simulink model "hw2_DCM_constant_flux"  (R2022a)
settings: Solver=ode45  StartTime=0.0  StopTime=10  MaxStep=0.0001  RelTol=1e-3  EnableMultiTasking=on
values from neighbouring files (symbols this model uses):
  Fv = 0.01 + N/3000    (= 0.0236666666667)    [hw2.m]    (also in hw3.m)
  J = 0.46    [hw2.m]    (also in hw3.m)
  kfi = M/In    (= 4.56074766355)    [hw2.m]    (also in hw3.m)
  La = 0.007    [hw2.m]    (also in hw3.m = 0.0007)
  Ra = 0.578    [hw2.m]    (also in hw3.m)
undefined symbols (not defined in the file or in its folder): sigbuilder_block
libraries: simulink x2
settings Model: Creator=user  LastModifiedBy=geote
settings SolverCC: AlgebraicLoopSolver=TrustRegion
settings DataIOCC: LimitDataPoints=on  SaveFormat=Array  SignalLoggingSaveFormat=ModelDataLogs  ReturnWorkspaceOutputs=off  SignalLoggingName=sigsOut
settings OptimizationCC: ExpressionDepthLimit=2147483647  InitFltsAndDblsToZero=on  LifeSpan=inf
settings DebuggingCC: SaveWithParameterizedLinksMsg=none  UnderspecifiedInitializationDetection=Classic  MergeDetectMultiDrivingBlocksExec=none  SignalResolutionControl=TryResolveAllWithWarning  MultiTaskDSMMsg=warning  MultiTaskCondExecSysMsg=none  FcnCallInpInsideContextMsg=warning  UnconnectedInputMsg=warning  UnconnectedOutputMsg=warning  UnconnectedLineMsg=warning  StateNameClashWarn=warning  SFUnexpectedBacktrackingDiag=warning  SFNoUnconditionalDefaultTransitionDiag=warning  SFMachineParentedDataDiag=warning  ArithmeticOperatorsInVariantConditions=warning
settings HardwareCC: ProdBitPerPointer=32  ProdBitPerSizeT=32  ProdBitPerPtrDiffT=32  ProdLargestAtomicFloat=None  ProdIntDivRoundTo=Undefined  ProdEndianess=Unspecified  ProdWordSize=32  ProdHWDeviceType=32-bit Generic  TargetUnknown=on
settings ModelReferenceCC: PropagateSignalLabelsOutOfModel=off
settings SFSimCC: SimUseLocalCustomCode=off  CustomCodeUndefinedFunction=UseInterfaceOnly
settings RTWCC: RTWUseLocalCustomCode=off
settings CodeAppCC: StateflowObjectComments=on
settings GRTTargetCC: TargetFcnLib=ansi_tfl_tmw.mat  TargetLangStandard=C89/C90 (ANSI)  CombineOutputUpdateFcns=off  GRTInterface=on
settings ConfigComp: CovMetricSettings=dw  CovSaveCumulativeToWorkspaceVar=on  CovSaveSingleToWorkspaceVar=on  CovExternalEMLEnable=off

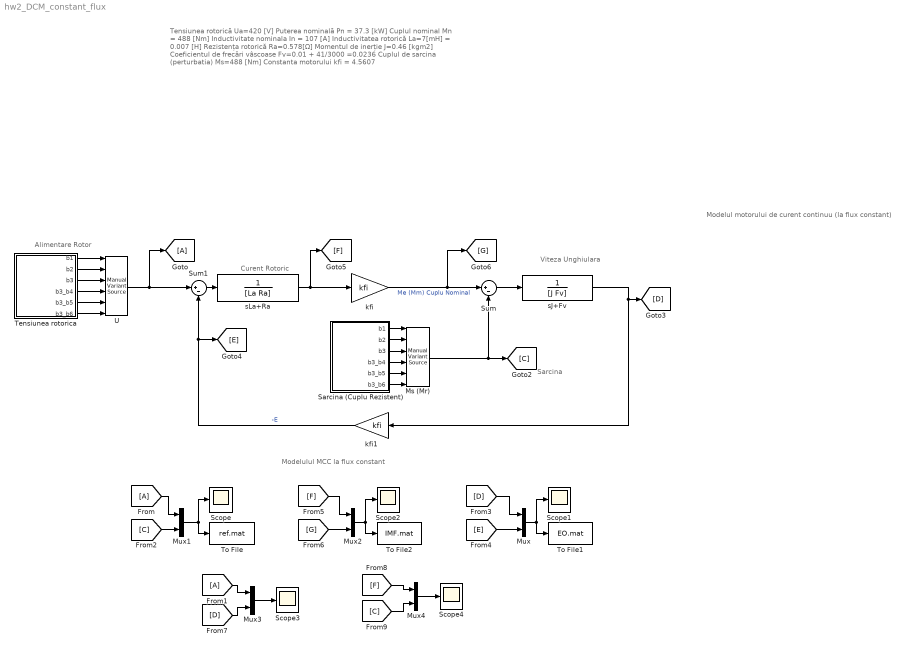
== system hw2_DCM_constant_flux ==
  note: Modelul motorului de curent continuu (la flux constant)
  note: Curent Rotoric
  note: Viteza
      | Unghiulara
  note: Modelulul MCC la flux constant
  note: Tensiunea rotorică Ua=420 [V]
      | Puterea nominală Pn = 37.3 [kW]
      |
      | Cuplul nominal Mn = 488 [Nm]
      | Inductivitate nominala In = 107 [A]
      |
      | Inductivitatea rotorică La=7[mH] = 0.007 [H]
      | Rezistența rotorică Ra=0.578[Ω]
      |
      | Momentul de inerție J=0.46 [kgm2]
      | Coeficientul de frecări vâscoase Fv=0.01 + 41/3000 =0.0236
      |
      | Cuplul de sarcina (perturbatia) Ms=488 [Nm]
      |
      | Constanta motorului kfi = 4.5607
  note: Alimentare Rotor
  note: Sarcina
  From : From
      settings: CloseFcn=tagdialog Close
  From1 : From
      settings: CloseFcn=tagdialog Close
  Goto : Goto
  Ms (Mr) : simulink/Signal Routing/Manual Variant Source  NumChoices=6  LabelModeActiveChoice=V_5
  Mux{,1..4} (5 alike) : Mux  Inputs=2
  Sarcina (Cuplu Rezistent) : Subsystem  Tag=STV Subsys  LoadFcn=sigbuilder_block('load');  StartFcn=sigbuilder_block('start');  StopFcn=sigbuilder_block('stop');  ClipboardFcn=sigbuilder_block('clipboard');  mask(Sigbuilder block){tuvar=[0:10]}
      mask help: Sigbuilder GUI
      mask init:
      | if ~strcmp(get_param(bdroot(gcbh),'SimulationStatus'),'stopped') tuvar = sigbuilder_block('maskInit'); end
      settings: CopyFcn=sigbuilder_block('copy');  DeleteFcn=sigbuilder_block('delete');  ModelCloseFcn=sigbuilder_block('modelClose');  PreSaveFcn=sigbuilder_block('preSave');  PauseFcn=sigbuilder_block('pause')  ContinueFcn=sigbuilder_block('continue')  NameChangeFcn=sigbuilder_block('namechange');  OpenFcn=sigbuilder_block('open',[412.2 7.8 574.8 510.6 ]);  CloseFcn=sigbuilder_block('close');
      mask Display: plot(0, 0, 100, 100,[2, 2, 32, 32, 2], [68, 8, 8, 68, 68],[32, 2], [38, 38], [32, 19, 2],[53, 60, 44], [32, 17, 17, 2],[16, 16, 31, 31]);txt = getActiveGroup(gcbh);text(2, 100, txt,'verticalAlignment', 'top');
  Scope{,1..4} (5 alike) : Scope
  Sum : Sum  Inputs=|+-  SaturateOnIntegerOverflow=on
  Sum1 : Sum  Inputs=|+-  SaturateOnIntegerOverflow=on
  Tensiunea rotorica : Subsystem  Tag=STV Subsys  LoadFcn=sigbuilder_block('load');  StartFcn=sigbuilder_block('start');  StopFcn=sigbuilder_block('stop');  ClipboardFcn=sigbuilder_block('clipboard');  mask(Sigbuilder block){tuvar=[0:10]}
      mask help: Sigbuilder GUI
      mask init:
      | if ~strcmp(get_param(bdroot(gcbh),'SimulationStatus'),'stopped') tuvar = sigbuilder_block('maskInit'); end
      settings: CopyFcn=sigbuilder_block('copy');  DeleteFcn=sigbuilder_block('delete');  ModelCloseFcn=sigbuilder_block('modelClose');  PreSaveFcn=sigbuilder_block('preSave');  PauseFcn=sigbuilder_block('pause')  ContinueFcn=sigbuilder_block('continue')  NameChangeFcn=sigbuilder_block('namechange');  OpenFcn=sigbuilder_block('open',[0.6 36.6 574.8 549.6 ]);  CloseFcn=sigbuilder_block('close');
      mask Display: plot(0, 0, 100, 100,[2, 2, 32, 32, 2], [68, 8, 8, 68, 68],[32, 2], [38, 38], [32, 19, 2],[53, 60, 44], [32, 17, 17, 2],[16, 16, 31, 31]);txt = getActiveGroup(gcbh);text(2, 100, txt,'verticalAlignment', 'top');
  To File : ToFile  Filename=ref.mat  MatrixName=ref
  To File1 : ToFile  Filename=EO.mat  MatrixName=EO
  To File2 : ToFile  Filename=IMF.mat  MatrixName=IMF
  U : simulink/Signal Routing/Manual Variant Source  NumChoices=6  LabelModeActiveChoice=V_5
  kfi : Gain  Gain=kfi  SaturateOnIntegerOverflow=on  OutDataTypeStr=Inherit: Same as input  ParamDataTypeStr=Inherit: Same as input
  kfi1 : Gain  Gain=kfi  SaturateOnIntegerOverflow=on  OutDataTypeStr=Inherit: Same as input  ParamDataTypeStr=Inherit: Same as input
  sJ+Fv : TransferFcn  Denominator=[J Fv]
  sLa+Ra : TransferFcn  Denominator=[La Ra]
  wires:
  Sum1/1 -> sLa+Ra/1
  sLa+Ra/1 -> [F], kfi/1
  kfi/1 -> [G], Sum/1  "Me (Mm) Cuplu Nominal"
  kfi1/1 -> Sum1/2, [E]  "-E"
  sJ+Fv/1 -> kfi1/1, [D]
  Sum/1 -> sJ+Fv/1
  Mux/1 -> Scope1/1, To File1/1
  Mux2/1 -> To File2/1, Scope2/1
  Mux1/1 -> Scope/1, To File/1
  From/1 -> Mux1/1
  [C] -> Mux1/2
  [D] -> Mux/1
  [E] -> Mux/2
  [F] -> Mux2/1
  [G] -> Mux2/2
  U/1 -> Sum1/1, Goto/1
  Ms (Mr)/1 -> Sum/2, [C]
  Tensiunea rotorica/1(b1) -> U/1
  Tensiunea rotorica/2(b2) -> U/2
  Tensiunea rotorica/3(b3) -> U/3
  Tensiunea rotorica/4(b3_b4) -> U/4
  Tensiunea rotorica/5(b3_b5) -> U/5
  Tensiunea rotorica/6(b3_b6) -> U/6
  Mux3/1 -> Scope3/1
  [D] -> Mux3/2
  From1/1 -> Mux3/1
  [C] -> Mux4/2
  [F] -> Mux4/1
  Mux4/1 -> Scope4/1
  Sarcina (Cuplu Rezistent)/1(b1) -> Ms (Mr)/1
  Sarcina (Cuplu Rezistent)/2(b2) -> Ms (Mr)/2
  Sarcina (Cuplu Rezistent)/3(b3) -> Ms (Mr)/3
  Sarcina (Cuplu Rezistent)/4(b3_b4) -> Ms (Mr)/4
  Sarcina (Cuplu Rezistent)/5(b3_b5) -> Ms (Mr)/5
  Sarcina (Cuplu Rezistent)/6(b3_b6) -> Ms (Mr)/6

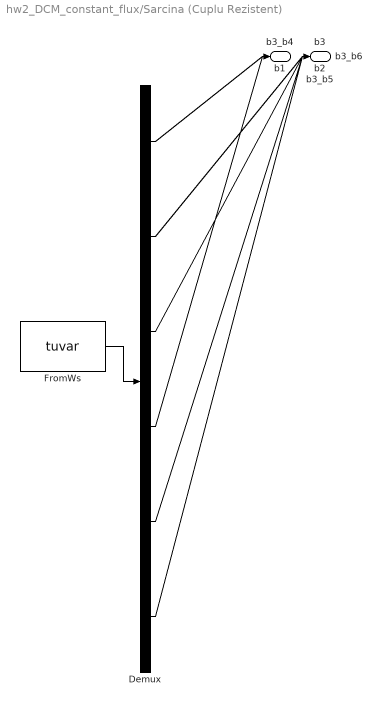
== system hw2_DCM_constant_flux/Sarcina (Cuplu Rezistent) ==
  Demux : Demux  Tag=STV Demux  Outputs=6
      settings: DisplayOption=none
  FromWs : FromWorkspace  Tag=STV FromWs  VariableName=tuvar
      SigBuilderData=|
      | common.afterFinalStr = 'Extrapolate'
      | common.sampleTime = 0
      | dataSet.timeRange = [0 10]
      | dataSet.name = 'Group 1'
      | sbobj.Groups.Name = 'Group 1'
      | sbobj.Groups.Signals(1).Name = 'b1'
      | sbobj.Groups.Signals(1).XData = [0 10]
      | sbobj.Groups.Signals(1).YData = [0 0]
      | sbobj.Groups.Signals(2).Name = 'b2'
      | sbobj.Groups.Signals(2).XData = [0 1 1 10]
      | sbobj.Groups.Signals(2).YData = [0 0 488 488]
      | sbobj.Groups.Signals(3).Name = 'b3'
      | sbobj.Groups.Signals(3).XData = [0 1 1 10]
      | sbobj.Groups.Signals(3).YData = [0 0 488 488]
      | sbobj.Groups.Signals(4).Name = 'b3_b4'
      | sbobj.Groups.Signals(4).XData = [0 1 1 10]
      | sbobj.Groups.Signals(4).YData = [0 0 488 488]
      | sbobj.Groups.Signals(5).Name = 'b3_b5'
      | sbobj.Groups.Signals(5).XData = [0 1 1 10]
      | sbobj.Groups.Signals(5).YData = [0 0 488 488]
      | sbobj.Groups.Signals(6).Name = 'b3_b6'
      | sbobj.Groups.Signals(6).XData = [0 1 1 4 4 5 5 6 6 10]
      | sbobj.Groups.Signals(6).YData = [0 0 488 488 244 244 488 488 732 740]
  b1 : Outport  Tag=STV Outport
  b2 : Outport  Tag=STV Outport  Port=2
  b3 : Outport  Tag=STV Outport  Port=3
  b3_b4 : Outport  Tag=STV Outport  Port=4
  b3_b5 : Outport  Tag=STV Outport  Port=5
  b3_b6 : Outport  Tag=STV Outport  Port=6
  wires:
  FromWs/1 -> Demux/1
  Demux/1 -> b1/1
  Demux/2 -> b2/1
  Demux/3 -> b3/1
  Demux/4 -> b3_b4/1
  Demux/5 -> b3_b5/1
  Demux/6 -> b3_b6/1

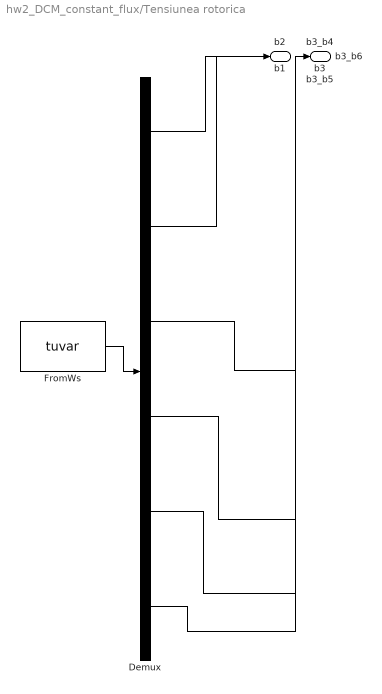
== system hw2_DCM_constant_flux/Tensiunea rotorica ==
  Demux : Demux  Tag=STV Demux  Outputs=6
      settings: DisplayOption=none
  FromWs : FromWorkspace  Tag=STV FromWs  VariableName=tuvar
      SigBuilderData=|
      | common.afterFinalStr = 'Extrapolate'
      | common.sampleTime = 0
      | dataSet.timeRange = [0 10]
      | dataSet.name = 'Group 1'
      | sbobj.Groups.Name = 'Group 1'
      | sbobj.Groups.Signals(1).Name = 'b1'
      | sbobj.Groups.Signals(1).XData = [0 1 1 10]
      | sbobj.Groups.Signals(1).YData = [0 0 420 420]
      | sbobj.Groups.Signals(2).Name = 'b2'
      | sbobj.Groups.Signals(2).XData = [0 1 1 10]
      | sbobj.Groups.Signals(2).YData = [0 0 420 420]
      | sbobj.Groups.Signals(3).Name = 'b3'
      | sbobj.Groups.Signals(3).XData = [0 1 2 10]
      | sbobj.Groups.Signals(3).YData = [0 0 420 420]
      | sbobj.Groups.Signals(4).Name = 'b3_b4'
      | sbobj.Groups.Signals(4).XData = [0 1 2 6.02 7 10]
      | sbobj.Groups.Signals(4).YData = [0 0 420 420 0 0]
      | sbobj.Groups.Signals(5).Name = 'b3_b5'
      | sbobj.Groups.Signals(5).XData = [0 1 2 6.02 8 10]
      | sbobj.Groups.Signals(5).YData = [0 0 420 420 -420 -420]
      | sbobj.Groups.Signals(6).Name = 'b3_b6'
      | sbobj.Groups.Signals(6).XData = [0 1 2 6.02 7.98 10]
      | sbobj.Groups.Signals(6).YData = [0 0 420 420 420 420]
  b1 : Outport  Tag=STV Outport
  b2 : Outport  Tag=STV Outport  Port=2
  b3 : Outport  Tag=STV Outport  Port=3
  b3_b4 : Outport  Tag=STV Outport  Port=4
  b3_b5 : Outport  Tag=STV Outport  Port=5
  b3_b6 : Outport  Tag=STV Outport  Port=6
  wires:
  FromWs/1 -> Demux/1
  Demux/1 -> b1/1
  Demux/2 -> b2/1
  Demux/3 -> b3/1
  Demux/4 -> b3_b4/1
  Demux/5 -> b3_b5/1
  Demux/6 -> b3_b6/1
